simulink model "assignment3EE311"  (R2019b)
settings: Solver=VariableStepAuto  StartTime=0.0  StopTime=10.0  RelTol=1e-3
libraries: dspadpt3 x2, dspsnks4 x1, dspsrcs4 x1
settings Model: Creator=hp  LastModifiedBy=hp

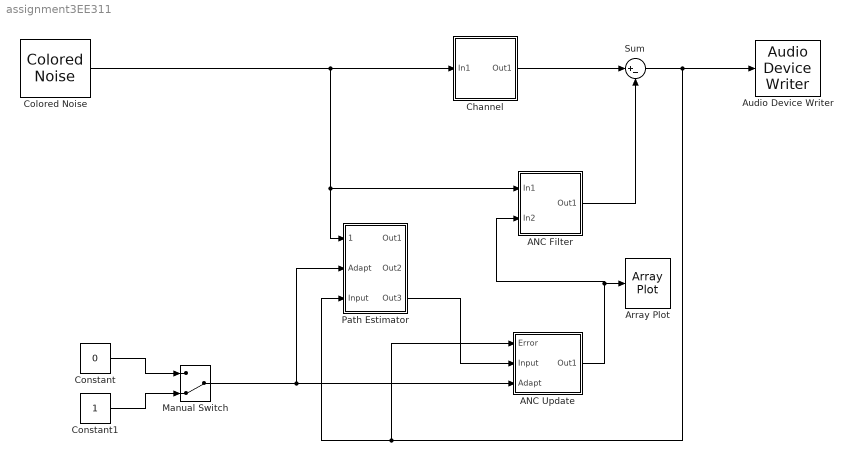
== system assignment3EE311 ==
  "ANC Filter " : Subsystem
  ANC Update : Subsystem
  Array Plot : ArrayPlot
  Audio Device Writer : dspsnks4/Audio Device Writer  Driver=DirectSound  Device=Default  InheritSampleRate=on  SampleRate=44100  BitDepth=16-bit integer  BufferSize=4096  NumBuffers=10  DefaultOutputChannelMapping=on  OutputChannelMapping=1:2  OutputNumUnderrunSamples=off  DriverIdx=1  DeviceWarnFlag=''
  "Channel " : Subsystem
  Colored Noise : dspsrcs4/Colored Noise  Color=pink  InverseFrequencyPower=1  BoundedOutput=off  NumChannels=1  OutputDataType=double  SamplesPerFrame=1  SampleTime=1/4000  RandomStream=mt19937ar with seed  Seed=67  SimulateUsing=Interpreted execution
      settings: SourceProductName=DSP System Toolbox  SourceProductBaseCode=DS
  Constant : Constant  Value=0
  Constant1 : Constant
  Manual Switch : ManualSwitch  CurrentSetting=0
  Path Estimator : Subsystem
  Sum : Sum  Inputs=|+-
  wires:
  Colored Noise/1 -> "Channel "/1(In1), Path Estimator/1(Desired), "ANC Filter "/1(In1)
  Sum/1 -> ANC Update/1("Error "), Path Estimator/3(Input), Audio Device Writer/1
  "ANC Filter "/1(Out1) -> Sum/2
  ANC Update/1(Out1) -> "ANC Filter "/2(In2), Array Plot/1
  "Channel "/1(Out1) -> Sum/1
  Constant/1 -> Manual Switch/1
  Constant1/1 -> Manual Switch/2
  Manual Switch/1 -> Path Estimator/2(Adapt), ANC Update/3("Adapt ")
  Path Estimator/3(Out3) -> ANC Update/2("Input ")

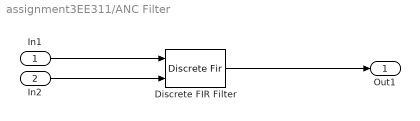
== system assignment3EE311/ANC Filter  ==
  In1 : Inport
  In2 : Inport  Port=2
  Discrete FIR Filter : DiscreteFir  CoefSource=Input port  InputProcessing=Columns as channels (frame based)
      settings: InputPortMap=u0,u1
  Out1 : Outport
  wires:
  In2/1 -> Discrete FIR Filter/2
  Discrete FIR Filter/1 -> Out1/1
  In1/1 -> Discrete FIR Filter/1

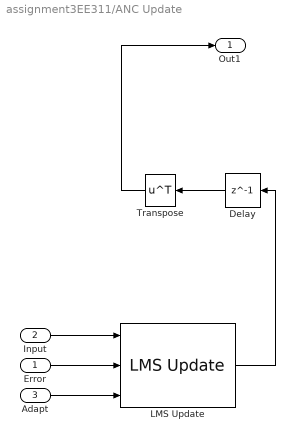
== system assignment3EE311/ANC Update ==
  "Error " : Inport
  "Input " : Inport  Port=2
  "Adapt " : Inport  Port=3
  Delay : Delay  DelayLength=1  InitialCondition=0
  LMS Update : dspadpt3/LMS Update  Method=Normalized LMS  Length=32  StepSizeSource=Property  StepSize=0.05  LeakageFactor=1.0  InitialConditions=0  EnableAdaptInput=on  EnableResetInput=off  SimulateUsing=Code generation
      settings: SourceProductName=DSP System Toolbox  SourceProductBaseCode=DS
  Transpose : Math  Operator=transpose  SignedPower=off  SaturateOnIntegerOverflow=on
  Out1 : Outport
  wires:
  Transpose/1 -> Out1/1
  "Input "/1 -> LMS Update/1
  "Error "/1 -> LMS Update/2
  Delay/1 -> Transpose/1
  LMS Update/1 -> Delay/1
  "Adapt "/1 -> LMS Update/3

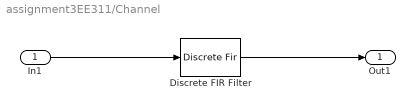
== system assignment3EE311/Channel  ==
  In1 : Inport
  Discrete FIR Filter : DiscreteFir  Coefficients=[0.5 0.3 1 0.3 -1 0.8 0.5 0.5]  InputProcessing=Columns as channels (frame based)
  Out1 : Outport
  wires:
  Discrete FIR Filter/1 -> Out1/1
  In1/1 -> Discrete FIR Filter/1

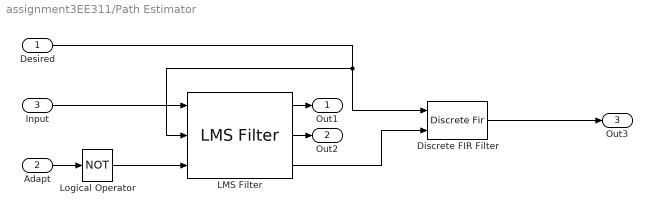
== system assignment3EE311/Path Estimator ==
  Desired : Inport
  Adapt : Inport  Port=2
  Input : Inport  Port=3
  Discrete FIR Filter : DiscreteFir  CoefSource=Input port  InputProcessing=Columns as channels (frame based)
      settings: InputPortMap=u0,u1
  LMS Filter : dspadpt3/LMS Filter  Algo=Normalized LMS  L=32  stepflag=Dialog  mu=0.05  leakage=1.0  ic=0  Adapt=on  resetflag=None  weights=on  addnparflag=off  roundingMode=Floor  overflowMode=off
      settings: SourceProductName=DSP System Toolbox  SourceProductBaseCode=DS
  Logical Operator : Logic  Operator=NOT  AllPortsSameDT=off  OutDataTypeStr=boolean
  Out1 : Outport
  Out2 : Outport  Port=2
  Out3 : Outport  Port=3
  wires:
  Discrete FIR Filter/1 -> Out3/1
  Input/1 -> LMS Filter/1
  LMS Filter/1 -> Out1/1
  LMS Filter/3 -> Discrete FIR Filter/2
  Desired/1 -> Discrete FIR Filter/1, LMS Filter/2
  LMS Filter/2 -> Out2/1
  Adapt/1 -> Logical Operator/1
  Logical Operator/1 -> LMS Filter/3
